simulink model "workingLR2"  (R2024a)
settings: Solver=VariableStepAuto  StartTime=0.0  StopTime=500  RelTol=1e-3
settings Model: Creator=Макс  LastModifiedBy=Григорий

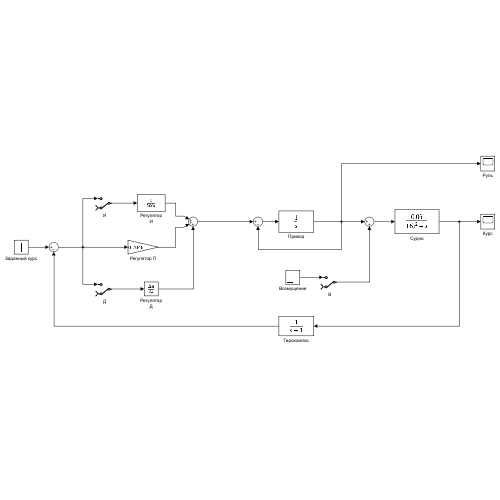
[thumbnail: Simulink's stored preview of the top-level diagram]
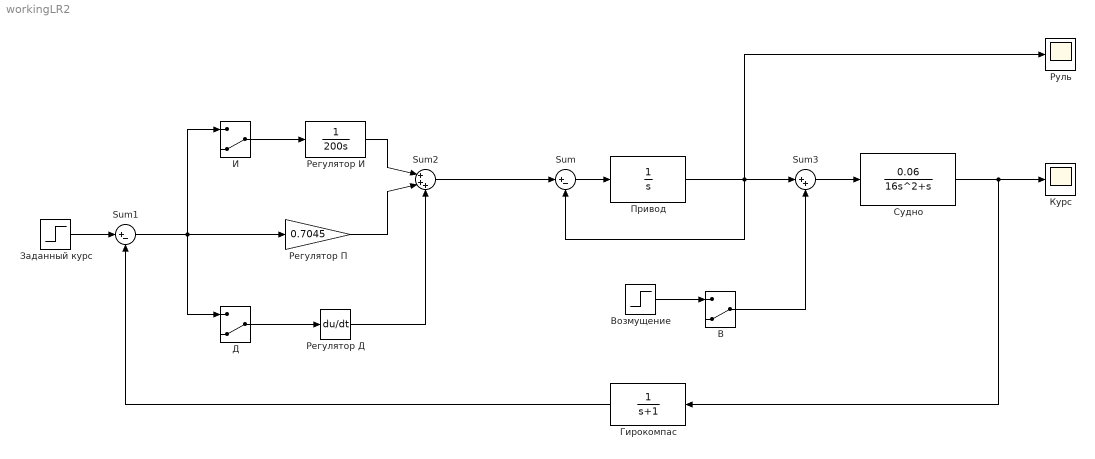
== system workingLR2 ==
  Sum : Sum  Inputs=|+-
  Sum1 : Sum  Inputs=|+-
  Sum2 : Sum  Inputs=|+++
  Sum3 : Sum  Inputs=|++
  В : ManualSwitch  CurrentSetting=0
  Возмущение : Step  Time=100  SampleTime=0
  Гирокомпас : TransferFcn  Denominator=[1 1]
  Д : ManualSwitch  CurrentSetting=0
  Заданный курс : Step  Time=0  After=10  SampleTime=0
  И : ManualSwitch  CurrentSetting=0
  Курс : Scope
  Привод : TransferFcn  Tag=Привод  Denominator=[1 0]
  Регулятор Д : Derivative
  Регулятор И : TransferFcn  Denominator=[200 0]
  Регулятор П : Gain  Gain=0.7045
  Руль : Scope
  Судно : TransferFcn  Numerator=[0.06]  Denominator=[16 1 0]
  wires:
  Регулятор И/1 -> Sum2/1
  Регулятор П/1 -> Sum2/2
  Регулятор Д/1 -> Sum2/3
  Заданный курс/1 -> Sum1/1
  Гирокомпас/1 -> Sum1/2
  Sum1/1 -> И/1, Д/1, Регулятор П/1
  И/1 -> Регулятор И/1
  Д/1 -> Регулятор Д/1
  Sum2/1 -> Sum/1
  Привод/1 -> Sum3/1, Sum/2, Руль/1
  Судно/1 -> Гирокомпас/1, Курс/1
  Sum/1 -> Привод/1
  Возмущение/1 -> В/1
  В/1 -> Sum3/2
  Sum3/1 -> Судно/1
